simulink model "PVModel3"  (R2023a)
settings: Solver=ode1  StartTime=0.0  StopTime=3.84  FixedStep=0.001  MaxStep=0.0748  RelTol=1e-3
values from neighbouring files (symbols this model uses):
  A = Aoff    [BoostConverterHybrid.m]    (also in PV_Params.mat = 1.3)
  Isc = 8.61    [PV_Params.mat]    (also in parameterEstimationv2.m = 5.45)
  Ki = 0.05    [PV_Params.mat]
  Kv = -0.32    [PV_Params.mat]
  Ns = 60    [PV_Params.mat]
  Rp = 415    [PV_Params.mat]    (also in battery_params_v2.m = 0.003103; parameterEstimationv2.m = R_p)
  Rs = 0.22    [PV_Params.mat]    (also in battery_params_v2.m = 0.010822; parameterEstimationv2.m = R_s)
  Voc = 38.41    [PV_Params.mat]    (also in parameterEstimationv2.m = 43.6)
libraries: SignalEditorBlockLib x1
settings Model: Creator=lucea  LastModifiedBy=gabrielcrisan

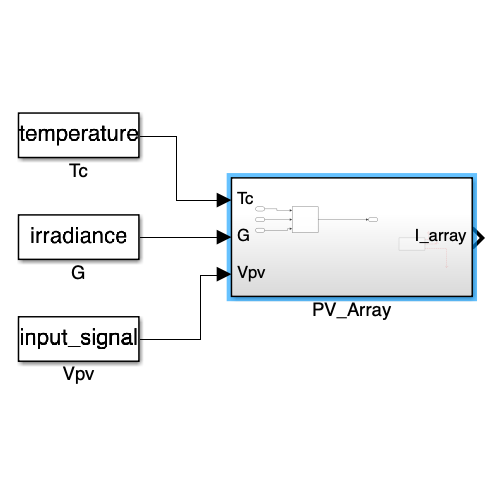
[thumbnail: Simulink's stored preview of the top-level diagram]
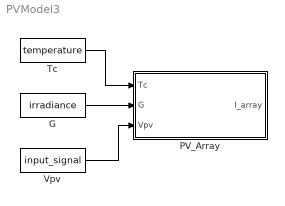
== system PVModel3 ==
  G : FromWorkspace  VariableName=irradiance
  PV_Array : Subsystem
  Tc : FromWorkspace  VariableName=temperature
  Vpv : FromWorkspace  VariableName=input_signal
  wires:
  Vpv/1 -> PV_Array/3(Vpv)
  G/1 -> PV_Array/2(G)
  Tc/1 -> PV_Array/1(Tc)

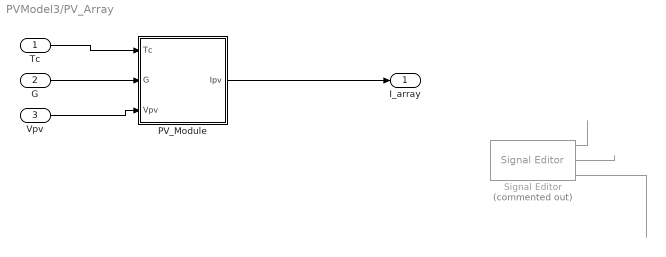
== system PVModel3/PV_Array ==
  Tc : Inport
  G : Inport  Port=2
  Vpv : Inport  Port=3
  PV_Module : Subsystem
  Signal Editor : SignalEditorBlockLib/Signal Editor  Commented=on  FileName=scenario1sigeditor.mat  ActiveScenario=Scenario  ActiveSignal=G  IsBus=off  OutputBusObjectStr=Bus: BusObject  SampleTime=-1  Interpolate=off  ZeroCross=off  OutputAfterFinalValue=Holding final value  Unit=inherit  PreserveSignalName=on  ApplySigPropsToAllScenarios=off
  I_array : Outport
  wires:
  G/1 -> PV_Module/2(G)
  Tc/1 -> PV_Module/1(Tc)
  Signal Editor/1 -> ?
  Signal Editor/2 -> ?
  Signal Editor/3 -> ?
  PV_Module/1(Ipv) -> I_array/1
  Vpv/1 -> PV_Module/3(Vpv)

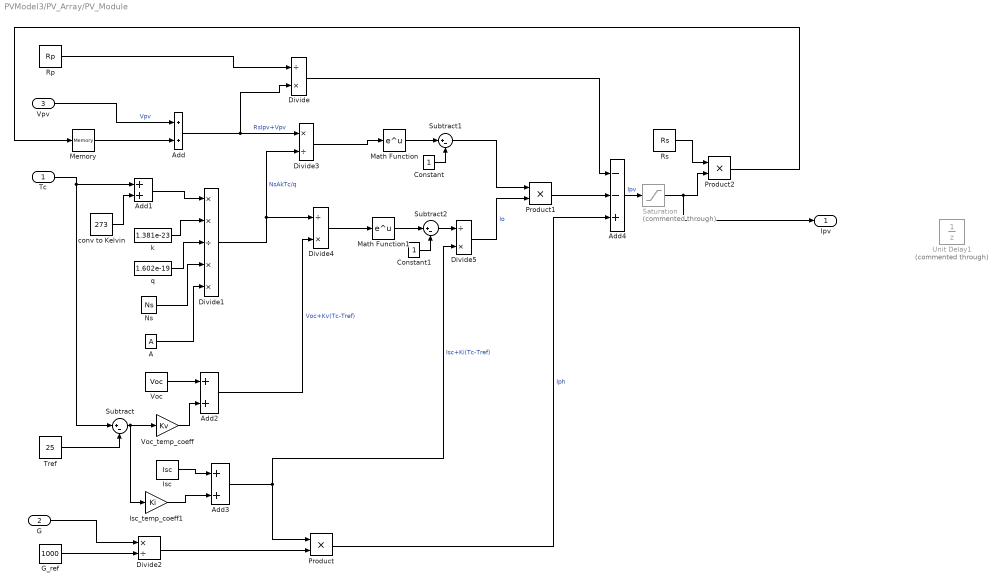
== system PVModel3/PV_Array/PV_Module ==
  Tc : Inport
  G : Inport  Port=2
  Vpv : Inport  Port=3
  A : Constant  Value=A
  Add{,1..3} (4 alike) : Sum
  Add4 : Sum  Inputs=--+
  Constant : Constant
  Constant1 : Constant
  Divide : Product  Inputs=/*
  Divide1 : Product  Inputs=**/**
  Divide2 : Product  Inputs=*/
  Divide3 : Product  Inputs=*/
  Divide4 : Product  Inputs=/*
  Divide5 : Product  Inputs=/*
  G_ref : Constant  Value=1000
  Isc : Constant  Value=Isc
  Isc_temp_coeff1 : Gain  Gain=Ki
  Math Function : Math
  Math Function1 : Math
  Memory : Memory  InheritSampleTime=on
  Ns : Constant  Value=Ns
  Product : Product
  Product1 : Product
  Product2 : Product
  Rp : Constant  Value=Rp
  Rs : Constant  Value=Rs
  Saturation : Saturate  Commented=through  UpperLimit=inf  LowerLimit=0
  Subtract : Sum  Inputs=|+-
  Subtract1 : Sum  Inputs=|+-
  Subtract2 : Sum  Inputs=|+-
  Tref : Constant  Value=25
  Unit Delay1 : UnitDelay  Commented=through  SampleTime=-1  HasFrameUpgradeWarning=on
  Voc : Constant  Value=Voc
  Voc_temp_coeff : Gain  Gain=Kv
  conv to Kelvin : Constant  Value=273
  k : Constant  Value=1.381e-23
  q : Constant  Value=1.602e-19
  Ipv : Outport
  wires:
  Add1/1 -> Divide1/1
  Product/1 -> Add4/3  "Iph"
  k/1 -> Divide1/2
  Vpv/1 -> Add/1  "Vpv"
  Constant/1 -> Subtract1/2
  Add/1 -> Divide/2, Divide3/1  "RsIpv+Vpv"
  Divide5/1 -> Product1/2  "Io"
  Tc/1 -> Subtract/1, Add1/1
  Add3/1 -> Divide5/2, Product/1  "Isc+Ki(Tc-Tref)"
  Constant1/1 -> Subtract2/2
  Subtract1/1 -> Product1/1
  Divide4/1 -> Math Function1/1
  Divide1/1 -> Divide4/1, Divide3/2  "NsAkTc/q"
  Math Function/1 -> Subtract1/1
  q/1 -> Divide1/3
  Isc/1 -> Add3/1
  Voc_temp_coeff/1 -> Add2/2
  A/1 -> Divide1/5
  Tref/1 -> Subtract/2
  G_ref/1 -> Divide2/2
  Add4/1 -> Saturation/1  "Ipv"
  conv to Kelvin/1 -> Add1/2
  G/1 -> Divide2/1
  Subtract/1 -> Isc_temp_coeff1/1, Voc_temp_coeff/1
  Rp/1 -> Divide/1
  Ns/1 -> Divide1/4
  Isc_temp_coeff1/1 -> Add3/2
  Voc/1 -> Add2/1
  Math Function1/1 -> Subtract2/1
  Add2/1 -> Divide4/2  "Voc+Kv(Tc-Tref)"
  Subtract2/1 -> Divide5/1
  Rs/1 -> Product2/1
  Divide2/1 -> Product/2
  Divide3/1 -> Math Function/1
  Memory/1 -> Add/2
  Saturation/1 -> Ipv/1, Product2/2
  Product2/1 -> Memory/1
  Divide/1 -> Add4/1
  Product1/1 -> Add4/2
